simulink model "SF015A_WhlImbRejctn"  (R2013b)
settings: Solver=FixedStepDiscrete  SolverMode=SingleTasking  StartTime=0.0  StopTime=1  FixedStep=0.002  RelTol=1e-3
values from neighbouring files (symbols this model uses):
  ACTIVBANDMAX_ULS_U32 = DataDict.Constant    [SF015A_WhlImbRejctn_DataDict.m]
  ADAPVFILMAX_ULS_F32 = DataDict.Constant    [SF015A_WhlImbRejctn_DataDict.m]
  ARCHGLBPRM_180OVERPI_ULS_F32 = DataDict.Constant    [SF015A_WhlImbRejctn_DataDict.m]
  ARCHGLBPRM_2MILLISEC_SEC_F32 = DataDict.Constant    [SF015A_WhlImbRejctn_DataDict.m]
  ARCHGLBPRM_2PI_ULS_F32 = DataDict.Constant    [SF015A_WhlImbRejctn_DataDict.m]
  ARCHGLBPRM_FLOATZEROTHD_ULS_F32 = DataDict.Constant    [SF015A_WhlImbRejctn_DataDict.m]
  ARCHGLBPRM_PI_ULS_F32 = DataDict.Constant    [SF015A_WhlImbRejctn_DataDict.m]
  ARCHGLBPRM_PIOVER180_ULS_F32 = DataDict.Constant    [SF015A_WhlImbRejctn_DataDict.m]
  ARCHGLBPRM_PIOVER2_ULS_F32 = DataDict.Constant    [SF015A_WhlImbRejctn_DataDict.m]
  CALMINSPERCOUNT_ULS_F32 = DataDict.Constant    [SF015A_WhlImbRejctn_DataDict.m]
  DURATIONDISABLE_CNT_U16 = DataDict.Constant    [SF015A_WhlImbRejctn_DataDict.m]
  FILTWHLSPDMAX_MOTRADPERSEC_F32 = DataDict.Constant    [SF015A_WhlImbRejctn_DataDict.m]
  MICROSECTOMILLISEC_ULS_F32 = DataDict.Constant    [SF015A_WhlImbRejctn_DataDict.m]
  MINSTOMILLISEC_ULS_F32 = DataDict.Constant    [SF015A_WhlImbRejctn_DataDict.m]
  NINETY_ULS_F32 = DataDict.Constant    [SF015A_WhlImbRejctn_DataDict.m]
  NODEBSTEP_CNT_U16 = DataDict.Constant    [SF015A_WhlImbRejctn_DataDict.m]
  NROFDLY_CNT_U08 = DataDict.Constant    [SF015A_WhlImbRejctn_DataDict.m]
  ONEHALF_ULS_F32 = DataDict.Constant    [SF015A_WhlImbRejctn_DataDict.m]
  ONEHUNDRED_ULS_F32 = DataDict.Constant    [SF015A_WhlImbRejctn_DataDict.m]
  ONEOVRTHREE_ULS_F32 = DataDict.Constant    [SF015A_WhlImbRejctn_DataDict.m]
  ONEOVRTWENTY_ULS_F32 = DataDict.Constant    [SF015A_WhlImbRejctn_DataDict.m]
  ONETHOUSAND_ULS_F32 = DataDict.Constant    [SF015A_WhlImbRejctn_DataDict.m]
  PEAKMAX_ULS_F32 = DataDict.Constant    [SF015A_WhlImbRejctn_DataDict.m]
  PEAKMIN_ULS_F32 = DataDict.Constant    [SF015A_WhlImbRejctn_DataDict.m]
  PHAADJMAX_ULS_F32 = DataDict.Constant    [SF015A_WhlImbRejctn_DataDict.m]
  PITIMESSAMPLETIME_ULS_F32 = DataDict.Constant    [SF015A_WhlImbRejctn_DataDict.m]
  STOREDMINSPERCOUNT_ULS_F32 = DataDict.Constant    [SF015A_WhlImbRejctn_DataDict.m]
  TWO_ULS_F32 = DataDict.Constant    [SF015A_WhlImbRejctn_DataDict.m]
  TWOOVRTHREE_ULS_F32 = DataDict.Constant    [SF015A_WhlImbRejctn_DataDict.m]
  WhlImbRejctnAdpvFac = DataDict.Calibration    [SF015A_WhlImbRejctn_DataDict.m]
  WhlImbRejctnAutScaEna = DataDict.Calibration    [SF015A_WhlImbRejctn_DataDict.m]
  WhlImbRejctnAutScaTar = DataDict.Calibration    [SF015A_WhlImbRejctn_DataDict.m]
  WhlImbRejctnCurrMgnSlewPerLoop = DataDict.Calibration    [SF015A_WhlImbRejctn_DataDict.m]
  WhlImbRejctnDcTrendFltRcvryDly = DataDict.Calibration    [SF015A_WhlImbRejctn_DataDict.m]
  WhlImbRejctnDcTrendFltRcvryNegStep = DataDict.Calibration    [SF015A_WhlImbRejctn_DataDict.m]
  WhlImbRejctnDcTrendFltRcvryPosStep = DataDict.Calibration    [SF015A_WhlImbRejctn_DataDict.m]
  WhlImbRejctnDcTrendFltRcvryThd = DataDict.Calibration    [SF015A_WhlImbRejctn_DataDict.m]
  WhlImbRejctnDcTrendTh2Tq = DataDict.Calibration    [SF015A_WhlImbRejctn_DataDict.m]
  WhlImbRejctnDcTrendThTq = DataDict.Calibration    [SF015A_WhlImbRejctn_DataDict.m]
  WhlImbRejctnDcTrendTi2Sec = DataDict.Calibration    [SF015A_WhlImbRejctn_DataDict.m]
  WhlImbRejctnDcTrendTiSec = DataDict.Calibration    [SF015A_WhlImbRejctn_DataDict.m]
  WhlImbRejctnEnaSlewPerLoop = DataDict.Calibration    [SF015A_WhlImbRejctn_DataDict.m]
  WhlImbRejctnFctEna = DataDict.Calibration    [SF015A_WhlImbRejctn_DataDict.m]
  WhlImbRejctnFrqDiagcAmpThd = DataDict.Calibration    [SF015A_WhlImbRejctn_DataDict.m]
  WhlImbRejctnFrqDiagcEna = DataDict.Calibration    [SF015A_WhlImbRejctn_DataDict.m]
  WhlImbRejctnFrqDiagcFltRcvryDly = DataDict.Calibration    [SF015A_WhlImbRejctn_DataDict.m]
  WhlImbRejctnFrqDiagcFltRcvryNegStep = DataDict.Calibration    [SF015A_WhlImbRejctn_DataDict.m]
  WhlImbRejctnFrqDiagcFltRcvryPosStep = DataDict.Calibration    [SF015A_WhlImbRejctn_DataDict.m]
  WhlImbRejctnFrqDiagcFltRcvryThd = DataDict.Calibration    [SF015A_WhlImbRejctn_DataDict.m]
  WhlImbRejctnFrqDiagcThd = DataDict.Calibration    [SF015A_WhlImbRejctn_DataDict.m]
  WhlImbRejctnFrqDiagcTout = DataDict.Calibration    [SF015A_WhlImbRejctn_DataDict.m]
  WhlImbRejctnFrqDiagcUgrPoleMgn = DataDict.Calibration    [SF015A_WhlImbRejctn_DataDict.m]
  WhlImbRejctnFrqScaTblX = DataDict.Calibration    [SF015A_WhlImbRejctn_DataDict.m]
  WhlImbRejctnMaxDurn = DataDict.Calibration    [SF015A_WhlImbRejctn_DataDict.m]
  WhlImbRejctnMaxMgn = DataDict.Calibration    [SF015A_WhlImbRejctn_DataDict.m]
  WhlImbRejctnMaxMgnFltNegStep = DataDict.Calibration    [SF015A_WhlImbRejctn_DataDict.m]
  WhlImbRejctnMaxMgnFltPosStep = DataDict.Calibration    [SF015A_WhlImbRejctn_DataDict.m]
  WhlImbRejctnMaxMgnFltRcvryDly = DataDict.Calibration    [SF015A_WhlImbRejctn_DataDict.m]
  WhlImbRejctnMaxMgnFltRcvryNegStep = DataDict.Calibration    [SF015A_WhlImbRejctn_DataDict.m]
  WhlImbRejctnMaxMgnFltRcvryPosStep = DataDict.Calibration    [SF015A_WhlImbRejctn_DataDict.m]
  WhlImbRejctnMaxMgnFltRcvryThd = DataDict.Calibration    [SF015A_WhlImbRejctn_DataDict.m]
  WhlImbRejctnMaxMgnFltThd = DataDict.Calibration    [SF015A_WhlImbRejctn_DataDict.m]
  WhlImbRejctnMgnEstimnDeltaSca = DataDict.Calibration    [SF015A_WhlImbRejctn_DataDict.m]
  WhlImbRejctnMgnEstimnDiThd = DataDict.Calibration    [SF015A_WhlImbRejctn_DataDict.m]
  WhlImbRejctnMgnEstimnEnaThd = DataDict.Calibration    [SF015A_WhlImbRejctn_DataDict.m]
  WhlImbRejctnMgnEstimnFrq = DataDict.Calibration    [SF015A_WhlImbRejctn_DataDict.m]
  WhlImbRejctnMgnEstimnFrqDelta = DataDict.Calibration    [SF015A_WhlImbRejctn_DataDict.m]
  WhlImbRejctnMgnEstimnLeak = DataDict.Calibration    [SF015A_WhlImbRejctn_DataDict.m]
  WhlImbRejctnRampDwnTi = DataDict.Calibration    [SF015A_WhlImbRejctn_DataDict.m]
  WhlImbRejctnScaCncl = DataDict.Calibration    [SF015A_WhlImbRejctn_DataDict.m]
  WhlImbRejctnUgrPoleMgn = DataDict.Calibration    [SF015A_WhlImbRejctn_DataDict.m]
  WhlImbRejctnVehSpdEna = DataDict.Calibration    [SF015A_WhlImbRejctn_DataDict.m]
  WhlImbRejctnWhlSpdCorrlnFltRcvryDly = DataDict.Calibration    [SF015A_WhlImbRejctn_DataDict.m]
  WhlImbRejctnWhlSpdCorrlnFltRcvryNegStep = DataDict.Calibration    [SF015A_WhlImbRejctn_DataDict.m]
  WhlImbRejctnWhlSpdCorrlnFltRcvryPosStep = DataDict.Calibration    [SF015A_WhlImbRejctn_DataDict.m]
  WhlImbRejctnWhlSpdCorrlnFltRcvryThd = DataDict.Calibration    [SF015A_WhlImbRejctn_DataDict.m]
  WhlImbRejctnWhlSpdCorrlnThd = DataDict.Calibration    [SF015A_WhlImbRejctn_DataDict.m]
  WhlImbRejctnWhlSpdCorrlnTi = DataDict.Calibration    [SF015A_WhlImbRejctn_DataDict.m]
  WIRCMDMAX_MOTNWTMTR_F32 = DataDict.Constant    [SF015A_WhlImbRejctn_DataDict.m]
  ZERO_ULS_F32 = DataDict.Constant    [SF015A_WhlImbRejctn_DataDict.m]
undefined symbols (not defined in the file or in its folder): Cntr, NtcNr1, NvmGetErrSts1, SigQlfr1, Sts, SysSt1
libraries: simulink x32, FixdToFloat x32, Fil x20, NxtrLim x15, NxtrNvM x12, NxtrAbslt x8, NxtrMath x7, NxtrMax x6, NxtrMin x4, FloatToFixd x2, LnrIntrpn x2, NxtrSign x1
(part 8 of 12)

== system SF015A_WhlImbRejctn/WhlImbRejctn/WhlImbRejctnPer2/Flt Recovery- DC Trend/ElapsedTime1/If true and last step not true elapsed time = 0 get reference time  ==
  Action Port : ActionPort  ActionType=elseif
  Constant : Constant  Value=0  OutDataTypeStr=single
  CopyRight2 : Subsystem  Description=|  mask(Copyright Information){none=on}
      | Copyright info block.                                               
      |                                                                     
      | Place copyright information at the top of every subsystem in design.
      mask prompts: none "No parameters"
      mask help: Place copyright information at the top of every subsystem in design.
      mask Display:
      | NxtrConf = 'Nexteer Confidential';
      | 
      | sys = bdroot; %handle for the current model ("system")
      | first = get_param(sys,'Created');
      | first = first(end-3:end);  %year is last four digits
      | 
      | last = get_param(sys,'LastModifiedDate');
      | if isempty(last)
      |     last = datestr(now,'yyyy');
      | else
      |     last = last(end-3:end);
      | end
      | 
      | if strcmp(first,last)
      |     fprintf('%s -- Copyright %s Nexteer',NxtrConf,first)
      | else
      |     fprintf('%s -- %s%s- %s Nexteer',NxtrConf,char(169),first,last)
      | end
  Data Store Write : DataStoreWrite  DataStoreName=DcTrendRefTiEnaLrng
  GetRefTmr100MicroSec32bit : Subsystem
  "SpanTi " : Outport
  wires:
  Constant/1 -> "SpanTi "/1
  GetRefTmr100MicroSec32bit/1(RefTmr) -> Data Store Write/1

== system SF015A_WhlImbRejctn/WhlImbRejctn/WhlImbRejctnPer2/Flt Recovery- DC Trend/Update Fault Status/CopyRight2 ==

== system SF015A_WhlImbRejctn/WhlImbRejctn/WhlImbRejctnPer2/Flt Recovery- DC Trend/Update Fault Status/Towards Failed ==
  PosStep : Inport
  Cnt : Inport  Port=2
  Thd : Inport  Port=3
  Action Port : ActionPort  ActionType=then
  Add : Sum
  CopyRight2 : Subsystem  Description=|  mask(Copyright Information){none=on}
      | Copyright info block.                                               
      |                                                                     
      | Place copyright information at the top of every subsystem in design.
      mask prompts: none "No parameters"
      mask help: Place copyright information at the top of every subsystem in design.
      mask Display:
      | NxtrConf = 'Nexteer Confidential';
      | 
      | sys = bdroot; %handle for the current model ("system")
      | first = get_param(sys,'Created');
      | first = first(end-3:end);  %year is last four digits
      | 
      | last = get_param(sys,'LastModifiedDate');
      | if isempty(last)
      |     last = datestr(now,'yyyy');
      | else
      |     last = last(end-3:end);
      | end
      | 
      | if strcmp(first,last)
      |     fprintf('%s -- Copyright %s Nexteer',NxtrConf,first)
      | else
      |     fprintf('%s -- %s%s- %s Nexteer',NxtrConf,char(169),first,last)
      | end
  Min_f32 : NxtrMin/Min_f32  SFunctionSpec=single y1 = Min_f32(single u1, single u2)
      settings: AttributesFormatString=%<Name>
  Out1 : Outport
  wires:
  PosStep/1 -> Add/1
  Cnt/1 -> Add/2
  Add/1 -> Min_f32/1
  Thd/1 -> Min_f32/2
  Min_f32/1 -> Out1/1

== system SF015A_WhlImbRejctn/WhlImbRejctn/WhlImbRejctnPer2/Flt Recovery- DC Trend/Update Fault Status/Towards Passed ==
  NegStep : Inport
  Cnt : Inport  Port=2
  Thd : Inport  Port=3
  Action Port : ActionPort  ActionType=else
  Add : Sum
  CopyRight2 : Subsystem  Description=|  mask(Copyright Information){none=on}
      | Copyright info block.                                               
      |                                                                     
      | Place copyright information at the top of every subsystem in design.
      mask prompts: none "No parameters"
      mask help: Place copyright information at the top of every subsystem in design.
      mask Display:
      | NxtrConf = 'Nexteer Confidential';
      | 
      | sys = bdroot; %handle for the current model ("system")
      | first = get_param(sys,'Created');
      | first = first(end-3:end);  %year is last four digits
      | 
      | last = get_param(sys,'LastModifiedDate');
      | if isempty(last)
      |     last = datestr(now,'yyyy');
      | else
      |     last = last(end-3:end);
      | end
      | 
      | if strcmp(first,last)
      |     fprintf('%s -- Copyright %s Nexteer',NxtrConf,first)
      | else
      |     fprintf('%s -- %s%s- %s Nexteer',NxtrConf,char(169),first,last)
      | end
  Max_f32 : NxtrMax/Max_f32  SFunctionSpec=single y1 = Max_f32(single u1, single u2)
      settings: AttributesFormatString=%<Name>
  Unary Minus : UnaryMinus
  Out1 : Outport
  wires:
  NegStep/1 -> Unary Minus/1
  Unary Minus/1 -> Add/1
  Cnt/1 -> Add/2
  Add/1 -> Max_f32/1
  Thd/1 -> Max_f32/2
  Max_f32/1 -> Out1/1

== system SF015A_WhlImbRejctn/WhlImbRejctn/WhlImbRejctnPer2/Flt Recovery- DC Trend/Update Fault Status/Update to Failed ==
  In1 : Inport
  Action Port : ActionPort  ActionType=then
  CopyRight2 : Subsystem  Description=|  mask(Copyright Information){none=on}
      | Copyright info block.                                               
      |                                                                     
      | Place copyright information at the top of every subsystem in design.
      mask prompts: none "No parameters"
      mask help: Place copyright information at the top of every subsystem in design.
      mask Display:
      | NxtrConf = 'Nexteer Confidential';
      | 
      | sys = bdroot; %handle for the current model ("system")
      | first = get_param(sys,'Created');
      | first = first(end-3:end);  %year is last four digits
      | 
      | last = get_param(sys,'LastModifiedDate');
      | if isempty(last)
      |     last = datestr(now,'yyyy');
      | else
      |     last = last(end-3:end);
      | end
      | 
      | if strcmp(first,last)
      |     fprintf('%s -- Copyright %s Nexteer',NxtrConf,first)
      | else
      |     fprintf('%s -- %s%s- %s Nexteer',NxtrConf,char(169),first,last)
      | end
  Out1 : Outport
  wires:
  In1/1 -> Out1/1

== system SF015A_WhlImbRejctn/WhlImbRejctn/WhlImbRejctnPer2/Flt Recovery- DC Trend/Update Fault Status/Update to Passed ==
  In1 : Inport
  Action Port : ActionPort  ActionType=elseif
  CopyRight2 : Subsystem  Description=|  mask(Copyright Information){none=on}
      | Copyright info block.                                               
      |                                                                     
      | Place copyright information at the top of every subsystem in design.
      mask prompts: none "No parameters"
      mask help: Place copyright information at the top of every subsystem in design.
      mask Display:
      | NxtrConf = 'Nexteer Confidential';
      | 
      | sys = bdroot; %handle for the current model ("system")
      | first = get_param(sys,'Created');
      | first = first(end-3:end);  %year is last four digits
      | 
      | last = get_param(sys,'LastModifiedDate');
      | if isempty(last)
      |     last = datestr(now,'yyyy');
      | else
      |     last = last(end-3:end);
      | end
      | 
      | if strcmp(first,last)
      |     fprintf('%s -- Copyright %s Nexteer',NxtrConf,first)
      | else
      |     fprintf('%s -- %s%s- %s Nexteer',NxtrConf,char(169),first,last)
      | end
  Out1 : Outport
  wires:
  In1/1 -> Out1/1

== system SF015A_WhlImbRejctn/WhlImbRejctn/WhlImbRejctnPer2/Flt Recovery- Freq Diag/ElapsedTime1/CopyRight2 ==

== system SF015A_WhlImbRejctn/WhlImbRejctn/WhlImbRejctnPer2/Flt Recovery- Freq Diag/ElapsedTime1/If not true elapsed time = 0 ==
  Action Port : ActionPort  ActionType=then
  Constant : Constant  Value=0  OutDataTypeStr=single
  CopyRight2 : Subsystem  Description=|  mask(Copyright Information){none=on}
      | Copyright info block.                                               
      |                                                                     
      | Place copyright information at the top of every subsystem in design.
      mask prompts: none "No parameters"
      mask help: Place copyright information at the top of every subsystem in design.
      mask Display:
      | NxtrConf = 'Nexteer Confidential';
      | 
      | sys = bdroot; %handle for the current model ("system")
      | first = get_param(sys,'Created');
      | first = first(end-3:end);  %year is last four digits
      | 
      | last = get_param(sys,'LastModifiedDate');
      | if isempty(last)
      |     last = datestr(now,'yyyy');
      | else
      |     last = last(end-3:end);
      | end
      | 
      | if strcmp(first,last)
      |     fprintf('%s -- Copyright %s Nexteer',NxtrConf,first)
      | else
      |     fprintf('%s -- %s%s- %s Nexteer',NxtrConf,char(169),first,last)
      | end
  SpanTi : Outport
  wires:
  Constant/1 -> SpanTi/1

== system SF015A_WhlImbRejctn/WhlImbRejctn/WhlImbRejctnPer2/Flt Recovery- Freq Diag/ElapsedTime1/If true and last step is true calculate elapsed time  ==
  Action Port : ActionPort  ActionType=else
  Constant1 : Constant  Value=MICROSECTOMILLISEC_ULS_F32
  CopyRight2 : Subsystem  Description=|  mask(Copyright Information){none=on}
      | Copyright info block.                                               
      |                                                                     
      | Place copyright information at the top of every subsystem in design.
      mask prompts: none "No parameters"
      mask help: Place copyright information at the top of every subsystem in design.
      mask Display:
      | NxtrConf = 'Nexteer Confidential';
      | 
      | sys = bdroot; %handle for the current model ("system")
      | first = get_param(sys,'Created');
      | first = first(end-3:end);  %year is last four digits
      | 
      | last = get_param(sys,'LastModifiedDate');
      | if isempty(last)
      |     last = datestr(now,'yyyy');
      | else
      |     last = last(end-3:end);
      | end
      | 
      | if strcmp(first,last)
      |     fprintf('%s -- Copyright %s Nexteer',NxtrConf,first)
      | else
      |     fprintf('%s -- %s%s- %s Nexteer',NxtrConf,char(169),first,last)
      | end
  Data Store Read : DataStoreRead  DataStoreName=FrqDiagcRefTiEnaLrng
  Divide : Product  Inputs=**
  FixdToFloat_f32_u32 : FixdToFloat/FixdToFloat_f32_u32  Param1=0
  GetTiSpan100MicroSec32bit : Subsystem
  SpanTi : Outport
  wires:
  Constant1/1 -> Divide/2
  Divide/1 -> SpanTi/1
  GetTiSpan100MicroSec32bit/1(TiSpan) -> FixdToFloat_f32_u32/1
  Data Store Read/1 -> GetTiSpan100MicroSec32bit/1(RefTmr)
  FixdToFloat_f32_u32/1 -> Divide/1

== system SF015A_WhlImbRejctn/WhlImbRejctn/WhlImbRejctnPer2/Flt Recovery- Freq Diag/ElapsedTime1/If true and last step not true elapsed time = 0 get reference time  ==
  Action Port : ActionPort  ActionType=elseif
  Constant : Constant  Value=0  OutDataTypeStr=single
  CopyRight2 : Subsystem  Description=|  mask(Copyright Information){none=on}
      | Copyright info block.                                               
      |                                                                     
      | Place copyright information at the top of every subsystem in design.
      mask prompts: none "No parameters"
      mask help: Place copyright information at the top of every subsystem in design.
      mask Display:
      | NxtrConf = 'Nexteer Confidential';
      | 
      | sys = bdroot; %handle for the current model ("system")
      | first = get_param(sys,'Created');
      | first = first(end-3:end);  %year is last four digits
      | 
      | last = get_param(sys,'LastModifiedDate');
      | if isempty(last)
      |     last = datestr(now,'yyyy');
      | else
      |     last = last(end-3:end);
      | end
      | 
      | if strcmp(first,last)
      |     fprintf('%s -- Copyright %s Nexteer',NxtrConf,first)
      | else
      |     fprintf('%s -- %s%s- %s Nexteer',NxtrConf,char(169),first,last)
      | end
  Data Store Write : DataStoreWrite  DataStoreName=FrqDiagcRefTiEnaLrng
  GetRefTmr100MicroSec32bit : Subsystem
  "SpanTi " : Outport
  wires:
  Constant/1 -> "SpanTi "/1
  GetRefTmr100MicroSec32bit/1(RefTmr) -> Data Store Write/1

== system SF015A_WhlImbRejctn/WhlImbRejctn/WhlImbRejctnPer2/Flt Recovery- Freq Diag/Update Fault Status/CopyRight2 ==

== system SF015A_WhlImbRejctn/WhlImbRejctn/WhlImbRejctnPer2/Flt Recovery- Freq Diag/Update Fault Status/Towards Failed ==
  PosStep : Inport
  Cnt : Inport  Port=2
  Thd : Inport  Port=3
  Action Port : ActionPort  ActionType=then
  Add : Sum
  CopyRight2 : Subsystem  Description=|  mask(Copyright Information){none=on}
      | Copyright info block.                                               
      |                                                                     
      | Place copyright information at the top of every subsystem in design.
      mask prompts: none "No parameters"
      mask help: Place copyright information at the top of every subsystem in design.
      mask Display:
      | NxtrConf = 'Nexteer Confidential';
      | 
      | sys = bdroot; %handle for the current model ("system")
      | first = get_param(sys,'Created');
      | first = first(end-3:end);  %year is last four digits
      | 
      | last = get_param(sys,'LastModifiedDate');
      | if isempty(last)
      |     last = datestr(now,'yyyy');
      | else
      |     last = last(end-3:end);
      | end
      | 
      | if strcmp(first,last)
      |     fprintf('%s -- Copyright %s Nexteer',NxtrConf,first)
      | else
      |     fprintf('%s -- %s%s- %s Nexteer',NxtrConf,char(169),first,last)
      | end
  Min_f32 : NxtrMin/Min_f32  SFunctionSpec=single y1 = Min_f32(single u1, single u2)
      settings: AttributesFormatString=%<Name>
  Out1 : Outport
  wires:
  PosStep/1 -> Add/1
  Cnt/1 -> Add/2
  Add/1 -> Min_f32/1
  Thd/1 -> Min_f32/2
  Min_f32/1 -> Out1/1

== system SF015A_WhlImbRejctn/WhlImbRejctn/WhlImbRejctnPer2/Flt Recovery- Freq Diag/Update Fault Status/Towards Passed ==
  NegStep : Inport
  Cnt : Inport  Port=2
  Thd : Inport  Port=3
  Action Port : ActionPort  ActionType=else
  Add : Sum
  CopyRight2 : Subsystem  Description=|  mask(Copyright Information){none=on}
      | Copyright info block.                                               
      |                                                                     
      | Place copyright information at the top of every subsystem in design.
      mask prompts: none "No parameters"
      mask help: Place copyright information at the top of every subsystem in design.
      mask Display:
      | NxtrConf = 'Nexteer Confidential';
      | 
      | sys = bdroot; %handle for the current model ("system")
      | first = get_param(sys,'Created');
      | first = first(end-3:end);  %year is last four digits
      | 
      | last = get_param(sys,'LastModifiedDate');
      | if isempty(last)
      |     last = datestr(now,'yyyy');
      | else
      |     last = last(end-3:end);
      | end
      | 
      | if strcmp(first,last)
      |     fprintf('%s -- Copyright %s Nexteer',NxtrConf,first)
      | else
      |     fprintf('%s -- %s%s- %s Nexteer',NxtrConf,char(169),first,last)
      | end
  Max_f32 : NxtrMax/Max_f32  SFunctionSpec=single y1 = Max_f32(single u1, single u2)
      settings: AttributesFormatString=%<Name>
  Unary Minus : UnaryMinus
  Out1 : Outport
  wires:
  NegStep/1 -> Unary Minus/1
  Unary Minus/1 -> Add/1
  Cnt/1 -> Add/2
  Add/1 -> Max_f32/1
  Thd/1 -> Max_f32/2
  Max_f32/1 -> Out1/1

== system SF015A_WhlImbRejctn/WhlImbRejctn/WhlImbRejctnPer2/Flt Recovery- Freq Diag/Update Fault Status/Update to Failed ==
  In1 : Inport
  Action Port : ActionPort  ActionType=then
  CopyRight2 : Subsystem  Description=|  mask(Copyright Information){none=on}
      | Copyright info block.                                               
      |                                                                     
      | Place copyright information at the top of every subsystem in design.
      mask prompts: none "No parameters"
      mask help: Place copyright information at the top of every subsystem in design.
      mask Display:
      | NxtrConf = 'Nexteer Confidential';
      | 
      | sys = bdroot; %handle for the current model ("system")
      | first = get_param(sys,'Created');
      | first = first(end-3:end);  %year is last four digits
      | 
      | last = get_param(sys,'LastModifiedDate');
      | if isempty(last)
      |     last = datestr(now,'yyyy');
      | else
      |     last = last(end-3:end);
      | end
      | 
      | if strcmp(first,last)
      |     fprintf('%s -- Copyright %s Nexteer',NxtrConf,first)
      | else
      |     fprintf('%s -- %s%s- %s Nexteer',NxtrConf,char(169),first,last)
      | end
  Out1 : Outport
  wires:
  In1/1 -> Out1/1

== system SF015A_WhlImbRejctn/WhlImbRejctn/WhlImbRejctnPer2/Flt Recovery- Freq Diag/Update Fault Status/Update to Passed ==
  In1 : Inport
  Action Port : ActionPort  ActionType=elseif
  CopyRight2 : Subsystem  Description=|  mask(Copyright Information){none=on}
      | Copyright info block.                                               
      |                                                                     
      | Place copyright information at the top of every subsystem in design.
      mask prompts: none "No parameters"
      mask help: Place copyright information at the top of every subsystem in design.
      mask Display:
      | NxtrConf = 'Nexteer Confidential';
      | 
      | sys = bdroot; %handle for the current model ("system")
      | first = get_param(sys,'Created');
      | first = first(end-3:end);  %year is last four digits
      | 
      | last = get_param(sys,'LastModifiedDate');
      | if isempty(last)
      |     last = datestr(now,'yyyy');
      | else
      |     last = last(end-3:end);
      | end
      | 
      | if strcmp(first,last)
      |     fprintf('%s -- Copyright %s Nexteer',NxtrConf,first)
      | else
      |     fprintf('%s -- %s%s- %s Nexteer',NxtrConf,char(169),first,last)
      | end
  Out1 : Outport
  wires:
  In1/1 -> Out1/1

== system SF015A_WhlImbRejctn/WhlImbRejctn/WhlImbRejctnPer2/Flt Recovery- Max Mag/ElapsedTime1/CopyRight2 ==

== system SF015A_WhlImbRejctn/WhlImbRejctn/WhlImbRejctnPer2/Flt Recovery- Max Mag/ElapsedTime1/If not true elapsed time = 0 ==
  Action Port : ActionPort  ActionType=then
  Constant : Constant  Value=0  OutDataTypeStr=single
  CopyRight2 : Subsystem  Description=|  mask(Copyright Information){none=on}
      | Copyright info block.                                               
      |                                                                     
      | Place copyright information at the top of every subsystem in design.
      mask prompts: none "No parameters"
      mask help: Place copyright information at the top of every subsystem in design.
      mask Display:
      | NxtrConf = 'Nexteer Confidential';
      | 
      | sys = bdroot; %handle for the current model ("system")
      | first = get_param(sys,'Created');
      | first = first(end-3:end);  %year is last four digits
      | 
      | last = get_param(sys,'LastModifiedDate');
      | if isempty(last)
      |     last = datestr(now,'yyyy');
      | else
      |     last = last(end-3:end);
      | end
      | 
      | if strcmp(first,last)
      |     fprintf('%s -- Copyright %s Nexteer',NxtrConf,first)
      | else
      |     fprintf('%s -- %s%s- %s Nexteer',NxtrConf,char(169),first,last)
      | end
  SpanTi : Outport
  wires:
  Constant/1 -> SpanTi/1

== system SF015A_WhlImbRejctn/WhlImbRejctn/WhlImbRejctnPer2/Flt Recovery- Max Mag/ElapsedTime1/If true and last step is true calculate elapsed time  ==
  Action Port : ActionPort  ActionType=else
  Constant1 : Constant  Value=MICROSECTOMILLISEC_ULS_F32
  CopyRight2 : Subsystem  Description=|  mask(Copyright Information){none=on}
      | Copyright info block.                                               
      |                                                                     
      | Place copyright information at the top of every subsystem in design.
      mask prompts: none "No parameters"
      mask help: Place copyright information at the top of every subsystem in design.
      mask Display:
      | NxtrConf = 'Nexteer Confidential';
      | 
      | sys = bdroot; %handle for the current model ("system")
      | first = get_param(sys,'Created');
      | first = first(end-3:end);  %year is last four digits
      | 
      | last = get_param(sys,'LastModifiedDate');
      | if isempty(last)
      |     last = datestr(now,'yyyy');
      | else
      |     last = last(end-3:end);
      | end
      | 
      | if strcmp(first,last)
      |     fprintf('%s -- Copyright %s Nexteer',NxtrConf,first)
      | else
      |     fprintf('%s -- %s%s- %s Nexteer',NxtrConf,char(169),first,last)
      | end
  Data Store Read : DataStoreRead  DataStoreName=MaxMgnRefTiEnaLrng
  Divide : Product  Inputs=**
  FixdToFloat_f32_u32 : FixdToFloat/FixdToFloat_f32_u32  Param1=0
  GetTiSpan100MicroSec32bit : Subsystem
  SpanTi : Outport
  wires:
  Constant1/1 -> Divide/2
  Divide/1 -> SpanTi/1
  GetTiSpan100MicroSec32bit/1(TiSpan) -> FixdToFloat_f32_u32/1
  Data Store Read/1 -> GetTiSpan100MicroSec32bit/1(RefTmr)
  FixdToFloat_f32_u32/1 -> Divide/1

== system SF015A_WhlImbRejctn/WhlImbRejctn/WhlImbRejctnPer2/Flt Recovery- Max Mag/ElapsedTime1/If true and last step not true elapsed time = 0 get reference time  ==
  Action Port : ActionPort  ActionType=elseif
  Constant : Constant  Value=0  OutDataTypeStr=single
  CopyRight2 : Subsystem  Description=|  mask(Copyright Information){none=on}
      | Copyright info block.                                               
      |                                                                     
      | Place copyright information at the top of every subsystem in design.
      mask prompts: none "No parameters"
      mask help: Place copyright information at the top of every subsystem in design.
      mask Display:
      | NxtrConf = 'Nexteer Confidential';
      | 
      | sys = bdroot; %handle for the current model ("system")
      | first = get_param(sys,'Created');
      | first = first(end-3:end);  %year is last four digits
      | 
      | last = get_param(sys,'LastModifiedDate');
      | if isempty(last)
      |     last = datestr(now,'yyyy');
      | else
      |     last = last(end-3:end);
      | end
      | 
      | if strcmp(first,last)
      |     fprintf('%s -- Copyright %s Nexteer',NxtrConf,first)
      | else
      |     fprintf('%s -- %s%s- %s Nexteer',NxtrConf,char(169),first,last)
      | end
  Data Store Write : DataStoreWrite  DataStoreName=MaxMgnRefTiEnaLrng
  GetRefTmr100MicroSec32bit : Subsystem
  "SpanTi " : Outport
  wires:
  Constant/1 -> "SpanTi "/1
  GetRefTmr100MicroSec32bit/1(RefTmr) -> Data Store Write/1

== system SF015A_WhlImbRejctn/WhlImbRejctn/WhlImbRejctnPer2/Flt Recovery- Max Mag/Update Fault Status/CopyRight2 ==

== system SF015A_WhlImbRejctn/WhlImbRejctn/WhlImbRejctnPer2/Flt Recovery- Max Mag/Update Fault Status/Towards Failed ==
  PosStep : Inport
  Cnt : Inport  Port=2
  Thd : Inport  Port=3
  Action Port : ActionPort  ActionType=then
  Add : Sum
  CopyRight2 : Subsystem  Description=|  mask(Copyright Information){none=on}
      | Copyright info block.                                               
      |                                                                     
      | Place copyright information at the top of every subsystem in design.
      mask prompts: none "No parameters"
      mask help: Place copyright information at the top of every subsystem in design.
      mask Display:
      | NxtrConf = 'Nexteer Confidential';
      | 
      | sys = bdroot; %handle for the current model ("system")
      | first = get_param(sys,'Created');
      | first = first(end-3:end);  %year is last four digits
      | 
      | last = get_param(sys,'LastModifiedDate');
      | if isempty(last)
      |     last = datestr(now,'yyyy');
      | else
      |     last = last(end-3:end);
      | end
      | 
      | if strcmp(first,last)
      |     fprintf('%s -- Copyright %s Nexteer',NxtrConf,first)
      | else
      |     fprintf('%s -- %s%s- %s Nexteer',NxtrConf,char(169),first,last)
      | end
  Min_f32 : NxtrMin/Min_f32  SFunctionSpec=single y1 = Min_f32(single u1, single u2)
      settings: AttributesFormatString=%<Name>
  Out1 : Outport
  wires:
  PosStep/1 -> Add/1
  Cnt/1 -> Add/2
  Add/1 -> Min_f32/1
  Thd/1 -> Min_f32/2
  Min_f32/1 -> Out1/1

== system SF015A_WhlImbRejctn/WhlImbRejctn/WhlImbRejctnPer2/Flt Recovery- Max Mag/Update Fault Status/Towards Passed ==
  NegStep : Inport
  Cnt : Inport  Port=2
  Thd : Inport  Port=3
  Action Port : ActionPort  ActionType=else
  Add : Sum
  CopyRight2 : Subsystem  Description=|  mask(Copyright Information){none=on}
      | Copyright info block.                                               
      |                                                                     
      | Place copyright information at the top of every subsystem in design.
      mask prompts: none "No parameters"
      mask help: Place copyright information at the top of every subsystem in design.
      mask Display:
      | NxtrConf = 'Nexteer Confidential';
      | 
      | sys = bdroot; %handle for the current model ("system")
      | first = get_param(sys,'Created');
      | first = first(end-3:end);  %year is last four digits
      | 
      | last = get_param(sys,'LastModifiedDate');
      | if isempty(last)
      |     last = datestr(now,'yyyy');
      | else
      |     last = last(end-3:end);
      | end
      | 
      | if strcmp(first,last)
      |     fprintf('%s -- Copyright %s Nexteer',NxtrConf,first)
      | else
      |     fprintf('%s -- %s%s- %s Nexteer',NxtrConf,char(169),first,last)
      | end
  Max_f32 : NxtrMax/Max_f32  SFunctionSpec=single y1 = Max_f32(single u1, single u2)
      settings: AttributesFormatString=%<Name>
  Unary Minus : UnaryMinus
  Out1 : Outport
  wires:
  NegStep/1 -> Unary Minus/1
  Unary Minus/1 -> Add/1
  Cnt/1 -> Add/2
  Add/1 -> Max_f32/1
  Thd/1 -> Max_f32/2
  Max_f32/1 -> Out1/1

== system SF015A_WhlImbRejctn/WhlImbRejctn/WhlImbRejctnPer2/Flt Recovery- Max Mag/Update Fault Status/Update to Failed ==
  In1 : Inport
  Action Port : ActionPort  ActionType=then
  CopyRight2 : Subsystem  Description=|  mask(Copyright Information){none=on}
      | Copyright info block.                                               
      |                                                                     
      | Place copyright information at the top of every subsystem in design.
      mask prompts: none "No parameters"
      mask help: Place copyright information at the top of every subsystem in design.
      mask Display:
      | NxtrConf = 'Nexteer Confidential';
      | 
      | sys = bdroot; %handle for the current model ("system")
      | first = get_param(sys,'Created');
      | first = first(end-3:end);  %year is last four digits
      | 
      | last = get_param(sys,'LastModifiedDate');
      | if isempty(last)
      |     last = datestr(now,'yyyy');
      | else
      |     last = last(end-3:end);
      | end
      | 
      | if strcmp(first,last)
      |     fprintf('%s -- Copyright %s Nexteer',NxtrConf,first)
      | else
      |     fprintf('%s -- %s%s- %s Nexteer',NxtrConf,char(169),first,last)
      | end
  Out1 : Outport
  wires:
  In1/1 -> Out1/1

== system SF015A_WhlImbRejctn/WhlImbRejctn/WhlImbRejctnPer2/Flt Recovery- Max Mag/Update Fault Status/Update to Passed ==
  In1 : Inport
  Action Port : ActionPort  ActionType=elseif
  CopyRight2 : Subsystem  Description=|  mask(Copyright Information){none=on}
      | Copyright info block.                                               
      |                                                                     
      | Place copyright information at the top of every subsystem in design.
      mask prompts: none "No parameters"
      mask help: Place copyright information at the top of every subsystem in design.
      mask Display:
      | NxtrConf = 'Nexteer Confidential';
      | 
      | sys = bdroot; %handle for the current model ("system")
      | first = get_param(sys,'Created');
      | first = first(end-3:end);  %year is last four digits
      | 
      | last = get_param(sys,'LastModifiedDate');
      | if isempty(last)
      |     last = datestr(now,'yyyy');
      | else
      |     last = last(end-3:end);
      | end
      | 
      | if strcmp(first,last)
      |     fprintf('%s -- Copyright %s Nexteer',NxtrConf,first)
      | else
      |     fprintf('%s -- %s%s- %s Nexteer',NxtrConf,char(169),first,last)
      | end
  Out1 : Outport
  wires:
  In1/1 -> Out1/1

== system SF015A_WhlImbRejctn/WhlImbRejctn/WhlImbRejctnPer2/Flt Recovery- WhlSpdCorr Diag/ElapsedTime1/CopyRight2 ==

== system SF015A_WhlImbRejctn/WhlImbRejctn/WhlImbRejctnPer2/Flt Recovery- WhlSpdCorr Diag/ElapsedTime1/If not true elapsed time = 0 ==
  Action Port : ActionPort  ActionType=then
  Constant : Constant  Value=0  OutDataTypeStr=single
  CopyRight2 : Subsystem  Description=|  mask(Copyright Information){none=on}
      | Copyright info block.                                               
      |                                                                     
      | Place copyright information at the top of every subsystem in design.
      mask prompts: none "No parameters"
      mask help: Place copyright information at the top of every subsystem in design.
      mask Display:
      | NxtrConf = 'Nexteer Confidential';
      | 
      | sys = bdroot; %handle for the current model ("system")
      | first = get_param(sys,'Created');
      | first = first(end-3:end);  %year is last four digits
      | 
      | last = get_param(sys,'LastModifiedDate');
      | if isempty(last)
      |     last = datestr(now,'yyyy');
      | else
      |     last = last(end-3:end);
      | end
      | 
      | if strcmp(first,last)
      |     fprintf('%s -- Copyright %s Nexteer',NxtrConf,first)
      | else
      |     fprintf('%s -- %s%s- %s Nexteer',NxtrConf,char(169),first,last)
      | end
  SpanTi : Outport
  wires:
  Constant/1 -> SpanTi/1

== system SF015A_WhlImbRejctn/WhlImbRejctn/WhlImbRejctnPer2/Flt Recovery- WhlSpdCorr Diag/ElapsedTime1/If true and last step is true calculate elapsed time  ==
  Action Port : ActionPort  ActionType=else
  Constant1 : Constant  Value=MICROSECTOMILLISEC_ULS_F32
  CopyRight2 : Subsystem  Description=|  mask(Copyright Information){none=on}
      | Copyright info block.                                               
      |                                                                     
      | Place copyright information at the top of every subsystem in design.
      mask prompts: none "No parameters"
      mask help: Place copyright information at the top of every subsystem in design.
      mask Display:
      | NxtrConf = 'Nexteer Confidential';
      | 
      | sys = bdroot; %handle for the current model ("system")
      | first = get_param(sys,'Created');
      | first = first(end-3:end);  %year is last four digits
      | 
      | last = get_param(sys,'LastModifiedDate');
      | if isempty(last)
      |     last = datestr(now,'yyyy');
      | else
      |     last = last(end-3:end);
      | end
      | 
      | if strcmp(first,last)
      |     fprintf('%s -- Copyright %s Nexteer',NxtrConf,first)
      | else
      |     fprintf('%s -- %s%s- %s Nexteer',NxtrConf,char(169),first,last)
      | end
  Data Store Read : DataStoreRead  DataStoreName=WhlSpdCorrlnDiagcRefTiEnaLrng
  Divide : Product  Inputs=**
  FixdToFloat_f32_u32 : FixdToFloat/FixdToFloat_f32_u32  Param1=0
  GetTiSpan100MicroSec32bit : Subsystem
  SpanTi : Outport
  wires:
  Constant1/1 -> Divide/2
  Divide/1 -> SpanTi/1
  GetTiSpan100MicroSec32bit/1(TiSpan) -> FixdToFloat_f32_u32/1
  Data Store Read/1 -> GetTiSpan100MicroSec32bit/1(RefTmr)
  FixdToFloat_f32_u32/1 -> Divide/1

== system SF015A_WhlImbRejctn/WhlImbRejctn/WhlImbRejctnPer2/Flt Recovery- WhlSpdCorr Diag/ElapsedTime1/If true and last step not true elapsed time = 0 get reference time  ==
  Action Port : ActionPort  ActionType=elseif
  Constant : Constant  Value=0  OutDataTypeStr=single
  CopyRight2 : Subsystem  Description=|  mask(Copyright Information){none=on}
      | Copyright info block.                                               
      |                                                                     
      | Place copyright information at the top of every subsystem in design.
      mask prompts: none "No parameters"
      mask help: Place copyright information at the top of every subsystem in design.
      mask Display:
      | NxtrConf = 'Nexteer Confidential';
      | 
      | sys = bdroot; %handle for the current model ("system")
      | first = get_param(sys,'Created');
      | first = first(end-3:end);  %year is last four digits
      | 
      | last = get_param(sys,'LastModifiedDate');
      | if isempty(last)
      |     last = datestr(now,'yyyy');
      | else
      |     last = last(end-3:end);
      | end
      | 
      | if strcmp(first,last)
      |     fprintf('%s -- Copyright %s Nexteer',NxtrConf,first)
      | else
      |     fprintf('%s -- %s%s- %s Nexteer',NxtrConf,char(169),first,last)
      | end
  Data Store Write : DataStoreWrite  DataStoreName=WhlSpdCorrlnDiagcRefTiEnaLrng
  GetRefTmr100MicroSec32bit : Subsystem
  "SpanTi " : Outport
  wires:
  Constant/1 -> "SpanTi "/1
  GetRefTmr100MicroSec32bit/1(RefTmr) -> Data Store Write/1

== system SF015A_WhlImbRejctn/WhlImbRejctn/WhlImbRejctnPer2/Flt Recovery- WhlSpdCorr Diag/Update Fault Status/CopyRight2 ==

== system SF015A_WhlImbRejctn/WhlImbRejctn/WhlImbRejctnPer2/Flt Recovery- WhlSpdCorr Diag/Update Fault Status/Towards Failed ==
  PosStep : Inport
  Cnt : Inport  Port=2
  Thd : Inport  Port=3
  Action Port : ActionPort  ActionType=then
  Add : Sum
  CopyRight2 : Subsystem  Description=|  mask(Copyright Information){none=on}
      | Copyright info block.                                               
      |                                                                     
      | Place copyright information at the top of every subsystem in design.
      mask prompts: none "No parameters"
      mask help: Place copyright information at the top of every subsystem in design.
      mask Display:
      | NxtrConf = 'Nexteer Confidential';
      | 
      | sys = bdroot; %handle for the current model ("system")
      | first = get_param(sys,'Created');
      | first = first(end-3:end);  %year is last four digits
      | 
      | last = get_param(sys,'LastModifiedDate');
      | if isempty(last)
      |     last = datestr(now,'yyyy');
      | else
      |     last = last(end-3:end);
      | end
      | 
      | if strcmp(first,last)
      |     fprintf('%s -- Copyright %s Nexteer',NxtrConf,first)
      | else
      |     fprintf('%s -- %s%s- %s Nexteer',NxtrConf,char(169),first,last)
      | end
  Min_f32 : NxtrMin/Min_f32  SFunctionSpec=single y1 = Min_f32(single u1, single u2)
      settings: AttributesFormatString=%<Name>
  Out1 : Outport
  wires:
  PosStep/1 -> Add/1
  Cnt/1 -> Add/2
  Add/1 -> Min_f32/1
  Thd/1 -> Min_f32/2
  Min_f32/1 -> Out1/1

== system SF015A_WhlImbRejctn/WhlImbRejctn/WhlImbRejctnPer2/Flt Recovery- WhlSpdCorr Diag/Update Fault Status/Towards Passed ==
  NegStep : Inport
  Cnt : Inport  Port=2
  Thd : Inport  Port=3
  Action Port : ActionPort  ActionType=else
  Add : Sum
  CopyRight2 : Subsystem  Description=|  mask(Copyright Information){none=on}
      | Copyright info block.                                               
      |                                                                     
      | Place copyright information at the top of every subsystem in design.
      mask prompts: none "No parameters"
      mask help: Place copyright information at the top of every subsystem in design.
      mask Display:
      | NxtrConf = 'Nexteer Confidential';
      | 
      | sys = bdroot; %handle for the current model ("system")
      | first = get_param(sys,'Created');
      | first = first(end-3:end);  %year is last four digits
      | 
      | last = get_param(sys,'LastModifiedDate');
      | if isempty(last)
      |     last = datestr(now,'yyyy');
      | else
      |     last = last(end-3:end);
      | end
      | 
      | if strcmp(first,last)
      |     fprintf('%s -- Copyright %s Nexteer',NxtrConf,first)
      | else
      |     fprintf('%s -- %s%s- %s Nexteer',NxtrConf,char(169),first,last)
      | end
  Max_f32 : NxtrMax/Max_f32  SFunctionSpec=single y1 = Max_f32(single u1, single u2)
      settings: AttributesFormatString=%<Name>
  Unary Minus : UnaryMinus
  Out1 : Outport
  wires:
  NegStep/1 -> Unary Minus/1
  Unary Minus/1 -> Add/1
  Cnt/1 -> Add/2
  Add/1 -> Max_f32/1
  Thd/1 -> Max_f32/2
  Max_f32/1 -> Out1/1

== system SF015A_WhlImbRejctn/WhlImbRejctn/WhlImbRejctnPer2/Flt Recovery- WhlSpdCorr Diag/Update Fault Status/Update to Failed ==
  In1 : Inport
  Action Port : ActionPort  ActionType=then
  CopyRight2 : Subsystem  Description=|  mask(Copyright Information){none=on}
      | Copyright info block.                                               
      |                                                                     
      | Place copyright information at the top of every subsystem in design.
      mask prompts: none "No parameters"
      mask help: Place copyright information at the top of every subsystem in design.
      mask Display:
      | NxtrConf = 'Nexteer Confidential';
      | 
      | sys = bdroot; %handle for the current model ("system")
      | first = get_param(sys,'Created');
      | first = first(end-3:end);  %year is last four digits
      | 
      | last = get_param(sys,'LastModifiedDate');
      | if isempty(last)
      |     last = datestr(now,'yyyy');
      | else
      |     last = last(end-3:end);
      | end
      | 
      | if strcmp(first,last)
      |     fprintf('%s -- Copyright %s Nexteer',NxtrConf,first)
      | else
      |     fprintf('%s -- %s%s- %s Nexteer',NxtrConf,char(169),first,last)
      | end
  Out1 : Outport
  wires:
  In1/1 -> Out1/1

== system SF015A_WhlImbRejctn/WhlImbRejctn/WhlImbRejctnPer2/Flt Recovery- WhlSpdCorr Diag/Update Fault Status/Update to Passed ==
  In1 : Inport
  Action Port : ActionPort  ActionType=elseif
  CopyRight2 : Subsystem  Description=|  mask(Copyright Information){none=on}
      | Copyright info block.                                               
      |                                                                     
      | Place copyright information at the top of every subsystem in design.
      mask prompts: none "No parameters"
      mask help: Place copyright information at the top of every subsystem in design.
      mask Display:
      | NxtrConf = 'Nexteer Confidential';
      | 
      | sys = bdroot; %handle for the current model ("system")
      | first = get_param(sys,'Created');
      | first = first(end-3:end);  %year is last four digits
      | 
      | last = get_param(sys,'LastModifiedDate');
      | if isempty(last)
      |     last = datestr(now,'yyyy');
      | else
      |     last = last(end-3:end);
      | end
      | 
      | if strcmp(first,last)
      |     fprintf('%s -- Copyright %s Nexteer',NxtrConf,first)
      | else
      |     fprintf('%s -- %s%s- %s Nexteer',NxtrConf,char(169),first,last)
      | end
  Out1 : Outport
  wires:
  In1/1 -> Out1/1

== system SF015A_WhlImbRejctn/WhlImbRejctn/WhlImbRejctnPer2/WIR Low Speed Diagnostics/MaxPersisDiag/CheckCompPersistence ==
  ActiveBand1 : Inport
  ActiveBand2 : Inport  Port=2
  ActiveBand3 : Inport  Port=3
  Constant1 : Constant  Value=WhlImbRejctnMaxDurn
  Constant15 : Constant  Value=0  OutDataTypeStr=boolean
  Constant3 : Constant  Value=DURATIONDISABLE_CNT_U16
  CopyRight2 : Subsystem  Description=|  mask(Copyright Information){none=on}
      | Copyright info block.                                               
      |                                                                     
      | Place copyright information at the top of every subsystem in design.
      mask prompts: none "No parameters"
      mask help: Place copyright information at the top of every subsystem in design.
      mask Display:
      | NxtrConf = 'Nexteer Confidential';
      | 
      | sys = bdroot; %handle for the current model ("system")
      | first = get_param(sys,'Created');
      | first = first(end-3:end);  %year is last four digits
      | 
      | last = get_param(sys,'LastModifiedDate');
      | if isempty(last)
      |     last = datestr(now,'yyyy');
      | else
      |     last = last(end-3:end);
      | end
      | 
      | if strcmp(first,last)
      |     fprintf('%s -- Copyright %s Nexteer',NxtrConf,first)
      | else
      |     fprintf('%s -- %s%s- %s Nexteer',NxtrConf,char(169),first,last)
      | end
  Data Type Conversion1 : DataTypeConversion  OutDataTypeStr=boolean
  If1 : If  IfExpression=u1
  Merge5 : Merge
  NoFault : Subsystem  RequirementInfo={} %GIDa_5cd6baa3_1788_47cc_9cc9_7c946c5076b5  TreatAsAtomicUnit=on
  Relational Operator1 : RelationalOperator  Operator=<=  OutDataTypeStr=boolean
  Subsystem : Subsystem
  Fault : Outport
  wires:
  Constant1/1 -> Relational Operator1/1
  Relational Operator1/1 -> If1/1
  Constant3/1 -> Relational Operator1/2
  If1/1 -> Subsystem/Action
  ActiveBand1/1 -> Subsystem/1(Band)
  ActiveBand2/1 -> Subsystem/2(Band2)
  ActiveBand3/1 -> Subsystem/3(Band3)
  Merge5/1 -> Fault/1
  Subsystem/1(Fault) -> Merge5/1
  Constant15/1 -> Data Type Conversion1/1
  NoFault/1(Output) -> Merge5/2
  If1/2 -> NoFault/Action
  Data Type Conversion1/1 -> NoFault/1(Input)
